simulink model "sim_task_3"  (R2024a)
settings: Solver=FixedStepAuto  StartTime=0.0  StopTime=10.0  FixedStep=1e-3  RelTol=1e-3
settings Model: Creator=alexe  LastModifiedBy=alexe

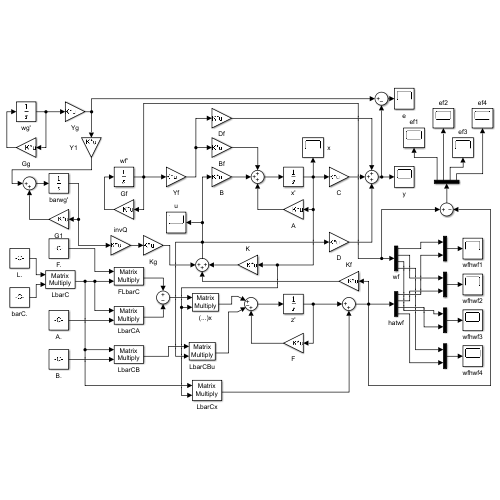
[thumbnail: Simulink's stored preview of the top-level diagram]
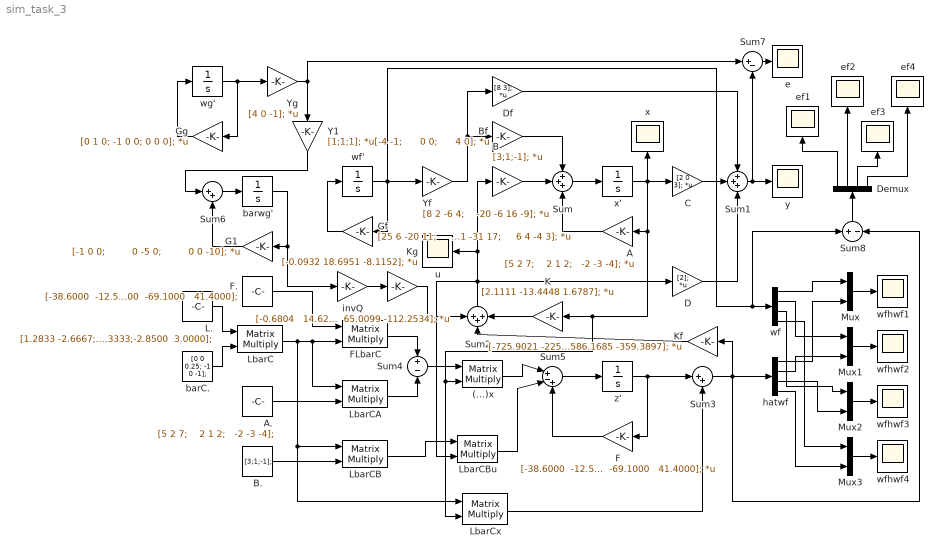
== system sim_task_3 ==
  (...)x : Product  Multiplication=Matrix(*)
  A : Gain  Gain=|  Multiplication=Matrix(K*u)
      | [5 2 7;
      |    2 1 2;
      |   -2 -3 -4];
  A. : Constant  Value=|  VectorParams1D=off
      | [5 2 7;
      |    2 1 2;
      |   -2 -3 -4];
  B : Gain  Gain=[3;1;-1];  Multiplication=Matrix(K*u)
  B. : Constant  Value=[3;1;-1];  VectorParams1D=off
  Bf : Gain  Gain=|  Multiplication=Matrix(K*u)
      | [-4 -1;
      |      0 0;
      |      4 0];
  C : Gain  Gain=[2 0 3];  Multiplication=Matrix(K*u)
  D : Gain  Gain=[2];  Multiplication=Matrix(K*u)
  Demux : Demux
  Df : Gain  Gain=[8 3];  Multiplication=Matrix(K*u)
  F : Gain  Gain=|  Multiplication=Matrix(K*u)
      | [-38.6000  -12.5667   30.3667  -18.1333;
      |    12.6000    0.3167   -6.6167    5.6333;
      |    12.6000    1.8167   -8.1167    5.6333;
      |    88.8000   27.7000  -69.1000   41.4000];
  F. : Constant  Value=|  VectorParams1D=off
      | [-38.6000  -12.5667   30.3667  -18.1333;
      |    12.6000    0.3167   -6.6167    5.6333;
      |    12.6000    1.8167   -8.1167    5.6333;
      |    88.8000   27.7000  -69.1000   41.4000];
  FLbarC : Product  Multiplication=Matrix(*)
  G1 : Gain  Gain=|  Multiplication=Matrix(K*u)
      | [-1 0 0;
      |         0 -5 0;
      |         0 0 -10];
  Gf : Gain  Gain=|  Multiplication=Matrix(K*u)
      | [25 6 -20 11;
      |     14 3 -10 4;
      |     40 11 -31 17;
      |     6 4 -4 3];
  Gg : Gain  Gain=[0 1 0; -1 0 0; 0 0 0];  Multiplication=Matrix(K*u)
  K : Gain  Gain=[2.1111 -13.4448 1.6787];  Multiplication=Matrix(K*u)
  Kf : Gain  Gain=[-725.9021 -225.1491 586.1685 -359.3897];  Multiplication=Matrix(K*u)
  Kg : Gain  Gain=[-0.0932 18.6951 -8.1152];  Multiplication=Matrix(K*u)
  L. : Constant  Value="[1.2833 -2.6667;-5.6583 -2.3333;-2.4083  -2.3333;-2.8500  3.0000];"  VectorParams1D=off
  LbarC : Product  Multiplication=Matrix(*)
  LbarCA : Product  Multiplication=Matrix(*)
  LbarCB : Product  Multiplication=Matrix(*)
  LbarCBu : Product  Multiplication=Matrix(*)
  LbarCx : Product  Multiplication=Matrix(*)
  Mux{,1..3} (4 alike) : Mux  Inputs=2
  Sum : Sum  Inputs=+++
  Sum1 : Sum  Inputs=+++
  Sum2 : Sum  Inputs=+++
  Sum3 : Sum  Inputs=|++
  Sum4 : Sum  Inputs=+|-
  Sum5 : Sum  Inputs=|+-+
  Sum6 : Sum  Inputs=|++
  Sum7 : Sum  Inputs=|+-
  Sum8 : Sum  Inputs=+-
  Y1 : Gain  Gain=[1;1;1];  Multiplication=Matrix(K*u)
  Yf : Gain  Gain=|  Multiplication=Matrix(K*u)
      | [8 2 -6 4;
      |    -20 -6 16 -9];
  Yg : Gain  Gain=[4 0 -1];  Multiplication=Matrix(K*u)
  barC. : Constant  Value="[0 0 0.25;   -1 0 -1];"  VectorParams1D=off
  barwg' : Integrator  InitialCondition=[0;0;0];
  e : Scope
  ef{1..4} (4 alike) : Scope
  hatwf : Demux
  invQ : Gain  Gain=|  Multiplication=Matrix(K*u)
      | [-0.6804   14.6291  -22.4543;
      |     0.2079  -17.8759   33.6724;
      |    -2.7766   65.0099 -112.2534];
  u : Scope
  wf : Demux
  wf' : Integrator  InitialCondition=[1;1;1;1];
  wfhwf{1..4} (4 alike) : Scope
  wg' : Integrator  InitialCondition=[0;1;1];
  x : Scope
  x' : Integrator  InitialCondition=[0;0;0];
  y : Scope
  z' : Integrator  InitialCondition=[0;0;0;0];
  wires:
  x'/1 -> x/1, C/1, LbarCx/2, (...)x/2, K/1, A/1
  Sum/1 -> x'/1
  A/1 -> Sum/3
  B/1 -> Sum/2
  Bf/1 -> Sum/1
  wf'/1 -> Gf/1, Sum8/1, wf/1, Yf/1
  Gf/1 -> wf'/1
  Yf/1 -> Df/1, Bf/1
  C/1 -> Sum1/2
  D/1 -> Sum1/3
  Df/1 -> Sum1/1
  K/1 -> Sum2/3
  z'/1 -> Sum3/1, F/1
  L./1 -> LbarC/1
  barC./1 -> LbarC/2
  LbarC/1 -> LbarCx/1, LbarCB/1, FLbarC/2, LbarCA/1
  F./1 -> FLbarC/1
  A./1 -> LbarCA/2
  FLbarC/1 -> Sum4/1
  LbarCA/1 -> Sum4/2
  Sum4/1 -> (...)x/1
  F/1 -> Sum5/3
  Sum5/1 -> z'/1
  (...)x/1 -> Sum5/1
  B./1 -> LbarCB/2
  LbarCB/1 -> LbarCBu/1
  LbarCBu/1 -> Sum5/2
  LbarCx/1 -> Sum3/2
  Kf/1 -> Sum2/2
  Sum3/1 -> Kf/1, Sum8/2, hatwf/1
  wg'/1 -> Yg/1, Gg/1
  Gg/1 -> wg'/1
  Yg/1 -> Sum7/1, Y1/1
  barwg'/1 -> invQ/1, G1/1
  Sum6/1 -> barwg'/1
  G1/1 -> Sum6/2
  Y1/1 -> Sum6/1
  invQ/1 -> Kg/1
  Kg/1 -> Sum2/1
  Sum2/1 -> LbarCBu/2, D/1, u/1, B/1
  Sum1/1 -> Sum7/2, y/1
  Sum7/1 -> e/1
  wf/1 -> Mux/1
  hatwf/1 -> Mux/2
  wf/2 -> Mux1/1
  hatwf/2 -> Mux1/2
  wf/3 -> Mux2/1
  hatwf/3 -> Mux2/2
  wf/4 -> Mux3/1
  hatwf/4 -> Mux3/2
  Mux/1 -> wfhwf1/1
  Mux1/1 -> wfhwf2/1
  Mux2/1 -> wfhwf3/1
  Mux3/1 -> wfhwf4/1
  Sum8/1 -> Demux/1
  Demux/1 -> ef1/1
  Demux/2 -> ef2/1
  Demux/3 -> ef3/1
  Demux/4 -> ef4/1
